simulink model "online_RLS_color_noise"  (R2017a)
settings: Solver=FixedStepDiscrete  StartTime=0.0  StopTime=1.49  FixedStep=0.01  RelTol=1e-3
settings Model: Creator=Lucci  LastModifiedBy=Lucci

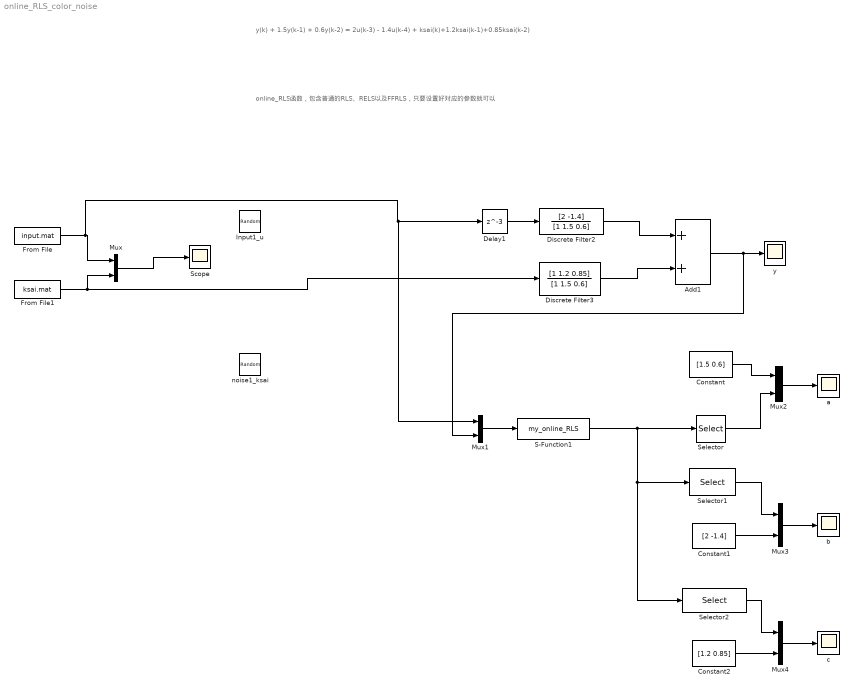
== system online_RLS_color_noise ==
  note: online_RLS函数，包含普通的RLS、RELS以及FFRLS，只要设置好对应的参数就可以
  note: y(k) + 1.5y(k-1) + 0.6y(k-2) = 2u(k-3) - 1.4u(k-4) + ksai(k)+1.2ksai(k-1)+0.85ksai(k-2)
  Add1 : Sum
  Constant : Constant  Value=[1.5 0.6]
  Constant1 : Constant  Value=[2 -1.4]
  Constant2 : Constant  Value=[1.2 0.85]
  Delay1 : Delay  DelayLength=3
  Discrete Filter2 : DiscreteFilter  Numerator=[2 -1.4]  Denominator=[1 1.5 0.6]
  Discrete Filter3 : DiscreteFilter  Numerator=[1 1.2 0.85]  Denominator=[1 1.5 0.6]
  From File : FromFile  FileName=input.mat  SampleTime=0
  From File1 : FromFile  FileName=ksai.mat  SampleTime=0
  Input1_u : RandomNumber  Seed=1  SampleTime=0.01
  Mux{,1..4} (5 alike) : Mux  Inputs=2
  S-Function1 : S-Function  FunctionName=my_online_RLS  Parameters=2,1,2,3,1  SFunctionDeploymentMode=off  EnableBusSupport=off
  Scope : Scope
  Selector : Selector  InputPortWidth=6  IndexOptions=Index vector (dialog)  Indices=[1 2]  OutputSizes=1
  Selector1 : Selector  InputPortWidth=6  IndexOptions=Index vector (dialog)  Indices=[3 4]  OutputSizes=1
  Selector2 : Selector  InputPortWidth=6  IndexOptions=Index vector (dialog)  Indices=[5 6]  OutputSizes=1
  a : Scope
  b : Scope
  c : Scope
  noise1_ksai : RandomNumber  Variance=0.8  Seed=1  SampleTime=0.01
  y : Scope
  wires:
  Mux1/1 -> S-Function1/1
  Add1/1 -> Mux1/2, y/1
  Discrete Filter2/1 -> Add1/1
  Delay1/1 -> Discrete Filter2/1
  Discrete Filter3/1 -> Add1/2
  Selector/1 -> Mux2/2
  Mux3/1 -> b/1
  Mux2/1 -> a/1
  Constant1/1 -> Mux3/2
  Selector1/1 -> Mux3/1
  Constant/1 -> Mux2/1
  S-Function1/1 -> Selector2/1, Selector1/1, Selector/1
  Constant2/1 -> Mux4/2
  Selector2/1 -> Mux4/1
  Mux4/1 -> c/1
  From File1/1 -> Discrete Filter3/1, Mux/2
  From File/1 -> Mux1/1, Delay1/1, Mux/1
  Mux/1 -> Scope/1
